simulink model "position_discrete"  (R2018b)
settings: Solver=VariableStepAuto  StartTime=0.0  StopTime=10  RelTol=1e-3
values from neighbouring files (symbols this model uses):
  Ad = sysd.A    [base_mix.m]
  Bd = sysd.B    [base_mix.m]
  Cd = sysd.C    [base_mix.m]
  Dd = sysd.D    [base_mix.m]
  Gd = Kfd(1)+Kfd(3)    [base_mix.m]
  Kfd = acker(Ad,Bd(:,1),Target_Pole_Discrete)    [base_mix.m]
libraries: cstblocks x1
settings Model: Creator=78224  LastModifiedBy=78224

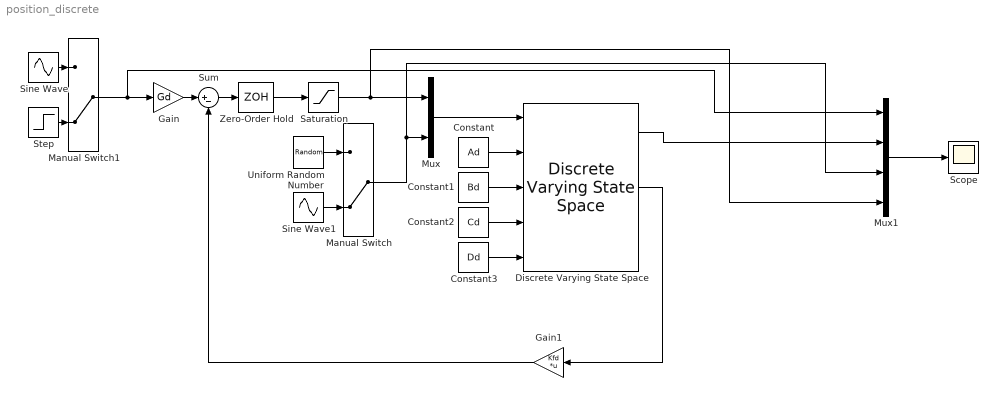
== system position_discrete ==
  Constant : Constant  Value=Ad  VectorParams1D=off
  Constant1 : Constant  Value=Bd  VectorParams1D=off
  Constant2 : Constant  Value=Cd  VectorParams1D=off
  Constant3 : Constant  Value=Dd  VectorParams1D=off
  Discrete Varying State Space : cstblocks/Linear Parameter Varying/Discrete Varying State Space  x0=0  Ts=0.01  OutputX=on  OutputDX=on
      settings: SourceProductName=Control System Toolbox  SourceProductBaseCode=CT
  Gain : Gain  Gain=Gd
  Gain1 : Gain  Gain=Kfd  Multiplication=Matrix(K*u)
  Manual Switch : ManualSwitch  CurrentSetting=0
  Manual Switch1 : ManualSwitch  CurrentSetting=0
  Mux : Mux  Inputs=2
  Mux1 : Mux
  Saturation : Saturate  UpperLimit=3.12  LowerLimit=-3.12
  Scope : Scope
  Sine Wave : Sin  Amplitude=60  Frequency=2*pi*0.2  SampleTime=0
  Sine Wave1 : Sin  Amplitude=0  Frequency=2*pi*0.2  SampleTime=0
  Step : Step  After=30  SampleTime=0
  Sum : Sum  Inputs=|+-
  Uniform Random Number : UniformRandomNumber  Minimum=-5  Maximum=5  SampleTime=0.2
  Zero-Order Hold : ZeroOrderHold  SampleTime=-1
  wires:
  Constant/1 -> Discrete Varying State Space/2
  Constant1/1 -> Discrete Varying State Space/3
  Constant2/1 -> Discrete Varying State Space/4
  Constant3/1 -> Discrete Varying State Space/5
  Mux1/1 -> Scope/1
  Mux/1 -> Discrete Varying State Space/1
  Manual Switch/1 -> Mux1/3, Mux/2
  Discrete Varying State Space/2 -> Gain1/1
  Gain/1 -> Sum/1
  Gain1/1 -> Sum/2
  Discrete Varying State Space/1 -> Mux1/2
  Uniform Random Number/1 -> Manual Switch/1
  Sine Wave1/1 -> Manual Switch/2
  Step/1 -> Manual Switch1/2
  Sine Wave/1 -> Manual Switch1/1
  Saturation/1 -> Mux1/4, Mux/1
  Manual Switch1/1 -> Gain/1, Mux1/1
  Zero-Order Hold/1 -> Saturation/1
  Sum/1 -> Zero-Order Hold/1
